simulink model "db5_2_Level_double"  (R2021a)
settings: Solver=VariableStepAuto  StartTime=0.0  StopTime=8  RelTol=1e-3
undefined symbols (not defined in the file): lambda2
libraries: dspsigops x5, dspquant2 x1
(part 1 of 2)
settings Model: Creator=Ruth Matienzo  LastModifiedBy=Ruth Matienzo

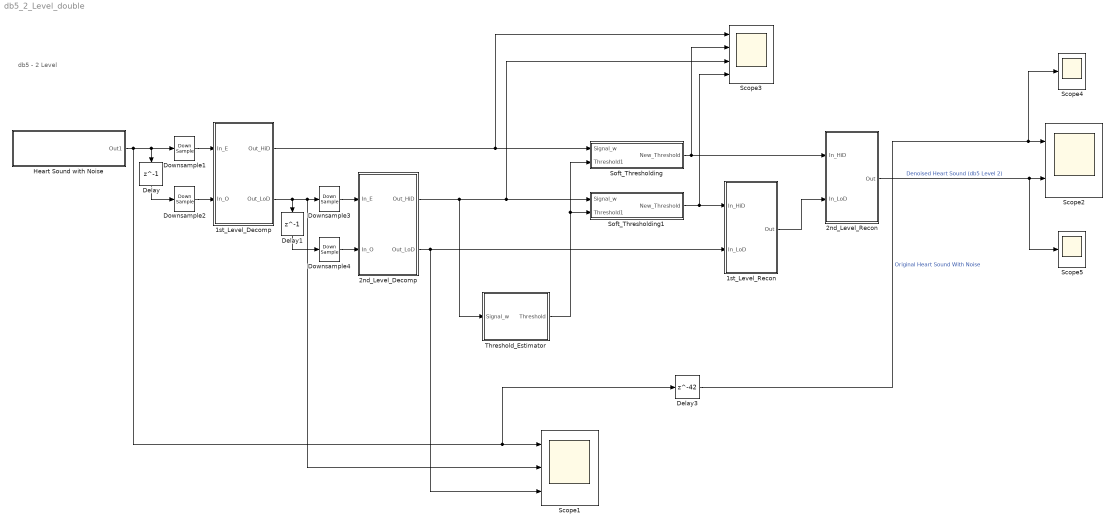
== system db5_2_Level_double ==
  note: db5 - 2 Level
  1st_Level_Decomp : Subsystem
  1st_Level_Recon : Subsystem
  2nd_Level_Decomp : Subsystem
  2nd_Level_Recon : Subsystem
  Delay : Delay  DelayLength=1  SampleTime=1/44100
  Delay1 : Delay  DelayLength=1  SampleTime=1/44100
  Delay3 : Delay  DelayLength=42  SampleTime=1/44100
  Downsample{1..4} (4 alike) : DownSample  N=30
  Heart Sound with Noise : Subsystem
  Scope1 : Scope  NumInputPorts=3
  Scope2 : Scope  NumInputPorts=2
  Scope3 : Scope  NumInputPorts=4
  Scope4 : Scope
  Scope5 : Scope
  Soft_Thresholding : Subsystem
  Soft_Thresholding1 : Subsystem
  Threshold_Estimator : Subsystem
  wires:
  1st_Level_Decomp/1(Out_HiD) -> Scope3/1, Soft_Thresholding/1(Signal_w)
  1st_Level_Recon/1(Out) -> 2nd_Level_Recon/2(In_LoD)
  Soft_Thresholding1/1(New_Threshold) -> 1st_Level_Recon/1(In_HiD), Scope3/4
  2nd_Level_Decomp/2(Out_LoD) -> 1st_Level_Recon/2(In_LoD), Scope1/3
  Downsample3/1 -> 2nd_Level_Decomp/1(In_E)
  2nd_Level_Decomp/1(Out_HiD) -> Threshold_Estimator/1(Signal_w), Scope3/3, Soft_Thresholding1/1(Signal_w)
  Downsample2/1 -> 1st_Level_Decomp/2(In_O)
  Delay1/1 -> Downsample4/1
  Heart Sound with Noise/1(Out1) -> Delay3/1, Scope1/1, Downsample1/1, Delay/1
  Downsample4/1 -> 2nd_Level_Decomp/2(In_O)
  Threshold_Estimator/1(Threshold) -> Soft_Thresholding1/2(Threshold1), Soft_Thresholding/2(Threshold1)
  Soft_Thresholding/1(New_Threshold) -> 2nd_Level_Recon/1(In_HiD), Scope3/2
  1st_Level_Decomp/2(Out_LoD) -> Scope1/2, Downsample3/1, Delay1/1
  Delay/1 -> Downsample2/1
  Downsample1/1 -> 1st_Level_Decomp/1(In_E)
  2nd_Level_Recon/1(Out) -> Scope5/1, Scope2/2  "Denoised Heart Sound (db5 Level 2)"
  Delay3/1 -> Scope4/1, Scope2/1  "Original Heart Sound With Noise"

== system db5_2_Level_double/1st_Level_Decomp ==
  In_E : Inport  OutDataTypeStr=double  SampleTime=1/44100
  In_O : Inport  Port=2  OutDataTypeStr=double  SampleTime=1/44100
  Add : Sum  AccumDataTypeStr=double  OutDataTypeStr=double
  Add1 : Sum  AccumDataTypeStr=double  OutDataTypeStr=double
  Delay1 : Delay  DelayLength=1  SampleTime=1/44100
  Delay2 : Delay  DelayLength=1  SampleTime=1/44100
  Divide1 : Product  Inputs=*/  OutDataTypeStr=double
  Divide2 : Product  Inputs=*/  OutDataTypeStr=double
  HiD : Constant  Value=1.216858059+0.784079501  OutDataTypeStr=double  SampleTime=1/44100
  HiD_Even : Subsystem
  HiD_Odd : Subsystem
  LoD : Constant  Value=0.784079501+1.216858059  OutDataTypeStr=double  SampleTime=1/44100
  LoD_Even : Subsystem
  LoD_Odd : Subsystem
  Out_HiD : Outport  OutDataTypeStr=double  SampleTime=1/44100
  Out_LoD : Outport  Port=2  OutDataTypeStr=double  SampleTime=1/44100
  wires:
  HiD/1 -> Divide1/2
  Add1/1 -> Divide2/1
  LoD/1 -> Divide2/2
  Add/1 -> Divide1/1
  Delay1/1 -> Out_HiD/1
  Divide1/1 -> Delay1/1
  Delay2/1 -> Out_LoD/1
  Divide2/1 -> Delay2/1
  In_E/1 -> LoD_Even/1(In_HiD_e), HiD_Even/1(In_HiD_e)
  HiD_Even/1(Out_HiD_e) -> Add/1
  In_O/1 -> LoD_Odd/1(In_HiD_e), HiD_Odd/1(In_HiD_e)
  HiD_Odd/1(Out_HiD_e) -> Add/2
  LoD_Even/1(Out_HiD_e) -> Add1/1
  LoD_Odd/1(Out_HiD_e) -> Add1/2

== system db5_2_Level_double/1st_Level_Recon ==
  In_HiD : Inport  OutDataTypeStr=double  SampleTime=1/44100
  In_LoD : Inport  Port=2  OutDataTypeStr=double  SampleTime=1/44100
  Add : Sum  AccumDataTypeStr=double  OutDataTypeStr=double
  Add1 : Sum  AccumDataTypeStr=double  OutDataTypeStr=double
  Add2 : Sum  AccumDataTypeStr=double  OutDataTypeStr=double
  Delay1 : Delay  DelayLength=1  SampleTime=1/44100
  Delay2 : Delay  DelayLength=1  SampleTime=1/44100
  Divide2 : Product  Inputs=*/  OutDataTypeStr=double  RndMeth=Zero  SaturateOnIntegerOverflow=on
  HiD1 : Constant  Value=0.707106781*1.41355  OutDataTypeStr=double  SampleTime=1/44100
  HiR_Even : Subsystem
  HiR_Odd : Subsystem
  LoR_Even : Subsystem
  LoR_Odd : Subsystem
  Rate Transition{,1..3} (4 alike) : RateTransition  OutPortSampleTime=1/44100
  Upsample : dspsigops/Upsample  N=30  phase=0  RateOptions=Allow multirate processing  ic=0  mode=Unused parameter value
  Upsample1 : dspsigops/Upsample  N=30  phase=0  RateOptions=Allow multirate processing  ic=0  mode=Unused parameter value
  Out : Outport  OutDataTypeStr=double  SampleTime=1/44100
  wires:
  In_HiD/1 -> HiR_Odd/1(In_HiR_o), HiR_Even/1(In_HiR_e)
  Add/1 -> Upsample1/1
  Add1/1 -> Upsample/1
  Upsample/1 -> Rate Transition/1
  Upsample1/1 -> Add2/1
  Delay2/1 -> Rate Transition1/1
  HiR_Even/1(Out_HiR_e) -> Add/1
  Rate Transition/1 -> Delay2/1
  Rate Transition1/1 -> Add2/2
  Rate Transition2/1 -> Delay1/1
  Delay1/1 -> Out/1
  HiD1/1 -> Rate Transition3/1
  Add2/1 -> Divide2/1
  Divide2/1 -> Rate Transition2/1
  Rate Transition3/1 -> Divide2/2
  In_LoD/1 -> LoR_Odd/1(In_LoR_o), LoR_Even/1(In_LoR_e)
  LoR_Even/1(Out_LoR_e) -> Add/2
  HiR_Odd/1(Out_HiR_o) -> Add1/1
  LoR_Odd/1(Out_LoR_o) -> Add1/2

== system db5_2_Level_double/2nd_Level_Decomp ==
  In_E : Inport  OutDataTypeStr=double  SampleTime=1/44100
  In_O : Inport  Port=2  OutDataTypeStr=double  SampleTime=1/44100
  Add : Sum  AccumDataTypeStr=double  OutDataTypeStr=double
  Add1 : Sum  AccumDataTypeStr=double  OutDataTypeStr=double
  Delay1 : Delay  DelayLength=1  SampleTime=1/44100
  Delay2 : Delay  DelayLength=1  SampleTime=1/44100
  Divide1 : Product  Inputs=*/  OutDataTypeStr=double
  Divide2 : Product  Inputs=*/  OutDataTypeStr=double
  HiD : Constant  Value=1.216858059+0.784079501  OutDataTypeStr=double  SampleTime=1/44100
  HiD_Even : Subsystem
  HiD_Odd : Subsystem
  LoD : Constant  Value=0.784079501+1.216858059  OutDataTypeStr=double  SampleTime=1/44100
  LoD_Even : Subsystem
  LoD_Odd : Subsystem
  Out_HiD : Outport  OutDataTypeStr=double  SampleTime=1/44100
  Out_LoD : Outport  Port=2  OutDataTypeStr=double  SampleTime=1/44100
  wires:
  HiD/1 -> Divide1/2
  Add1/1 -> Divide2/1
  LoD/1 -> Divide2/2
  Add/1 -> Divide1/1
  Delay1/1 -> Out_HiD/1
  Divide1/1 -> Delay1/1
  Delay2/1 -> Out_LoD/1
  Divide2/1 -> Delay2/1
  In_E/1 -> LoD_Even/1(In_HiD_e), HiD_Even/1(In_HiD_e)
  HiD_Even/1(Out_HiD_e) -> Add/1
  In_O/1 -> LoD_Odd/1(In_HiD_e), HiD_Odd/1(In_HiD_e)
  HiD_Odd/1(Out_HiD_e) -> Add/2
  LoD_Even/1(Out_HiD_e) -> Add1/1
  LoD_Odd/1(Out_HiD_e) -> Add1/2

== system db5_2_Level_double/2nd_Level_Recon ==
  In_HiD : Inport  OutDataTypeStr=double  SampleTime=1/44100
  In_LoD : Inport  Port=2  OutDataTypeStr=double  SampleTime=1/44100
  Add : Sum  AccumDataTypeStr=double  OutDataTypeStr=double
  Add1 : Sum  AccumDataTypeStr=double  OutDataTypeStr=double
  Add2 : Sum  AccumDataTypeStr=double  OutDataTypeStr=double
  Delay1 : Delay  DelayLength=1  SampleTime=1/44100
  Delay2 : Delay  DelayLength=1  SampleTime=1/44100
  Divide2 : Product  Inputs=*/  OutDataTypeStr=double  RndMeth=Zero  SaturateOnIntegerOverflow=on
  HiD1 : Constant  Value=0.707106781*1.41355  OutDataTypeStr=double  SampleTime=1/44100
  HiR_Even : Subsystem
  HiR_Odd : Subsystem
  LoR_Even : Subsystem
  LoR_Odd : Subsystem
  Rate Transition{,1..3} (4 alike) : RateTransition  OutPortSampleTime=1/44100
  Upsample : dspsigops/Upsample  N=30  phase=0  RateOptions=Allow multirate processing  ic=0  mode=Unused parameter value
  Upsample1 : dspsigops/Upsample  N=30  phase=0  RateOptions=Allow multirate processing  ic=0  mode=Unused parameter value
  Out : Outport  OutDataTypeStr=double  SampleTime=1/44100
  wires:
  In_HiD/1 -> HiR_Odd/1(In_HiR_o), HiR_Even/1(In_HiR_e)
  Add/1 -> Upsample1/1
  Add1/1 -> Upsample/1
  Upsample/1 -> Rate Transition/1
  Upsample1/1 -> Add2/1
  Delay2/1 -> Rate Transition1/1
  HiR_Even/1(Out_HiR_e) -> Add/1
  Rate Transition/1 -> Delay2/1
  Rate Transition1/1 -> Add2/2
  Rate Transition2/1 -> Delay1/1
  Delay1/1 -> Out/1
  HiD1/1 -> Rate Transition3/1
  Add2/1 -> Divide2/1
  Divide2/1 -> Rate Transition2/1
  Rate Transition3/1 -> Divide2/2
  In_LoD/1 -> LoR_Odd/1(In_LoR_o), LoR_Even/1(In_LoR_e)
  LoR_Even/1(Out_LoR_e) -> Add/2
  HiR_Odd/1(Out_HiR_o) -> Add1/1
  LoR_Odd/1(Out_LoR_o) -> Add1/2

== system db5_2_Level_double/Heart Sound with Noise ==
  Constant : Constant  Value=80000  OutDataTypeStr=double  SampleTime=1/44100
  Divide : Product  Inputs=*/  OutDataTypeStr=double
  From Workspace1 : FromWorkspace  VariableName=Audio_Heart_Noise  OutDataTypeStr=double  SampleTime=1/44100
  Gain2 : Gain  Gain=5  ParamDataTypeStr=double  OutDataTypeStr=double
  Pulse Generator : DiscretePulseGenerator  PulseType=Time based  Period=0.00022675736  PulseWidth=50
  Quantizer : Quantizer  QuantizationInterval=0.1
  Sample and Hold : dspsigops/Sample and Hold  trig=Rising edge  initCond=0  latchinput=off
  Uniform Encoder : dspquant2/Uniform Encoder  peak=2  bits=8  otype=Unsigned integer
  Out1 : Outport  OutDataTypeStr=double  SampleTime=1/44100
  wires:
  Sample and Hold/1 -> Quantizer/1
  Uniform Encoder/1 -> Divide/1
  Quantizer/1 -> Uniform Encoder/1
  Constant/1 -> Divide/2
  From Workspace1/1 -> Gain2/1
  Pulse Generator/1 -> Sample and Hold/Trigger
  Gain2/1 -> Sample and Hold/1
  Divide/1 -> Out1/1

== system db5_2_Level_double/Soft_Thresholding ==
  Signal_w : Inport  OutDataTypeStr=double  SampleTime=1/44100
  Threshold1 : Inport  Port=2  OutDataTypeStr=double  SampleTime=1/44100
  Abs : Abs  OutDataTypeStr=double
  Add1 : Sum  AccumDataTypeStr=double  OutDataTypeStr=double
  Constant : Constant  Value=0  OutDataTypeStr=double  SampleTime=1/44100
  Delay{1..7} (7 alike) : Delay  DelayLength=1  SampleTime=1/44100
  Divide : Product  Inputs=*/  OutDataTypeStr=double
  Gain1 : Gain  Gain=-1  ParamDataTypeStr=double  OutMin=-1  OutMax=-0.99  OutDataTypeStr=double
  Length : Constant  Value=lambda2  OutDataTypeStr=double  SampleTime=1/44100
  Relational Operator1 : RelationalOperator  Operator===  OutDataTypeStr=boolean  RndMeth=Simplest
  Relational Operator2 : RelationalOperator  Operator=>  OutDataTypeStr=boolean  RndMeth=Simplest
  Relational Operator3 : RelationalOperator  Operator=<  OutDataTypeStr=boolean  RndMeth=Simplest
  Relational Operator4 : RelationalOperator  Operator=>  OutDataTypeStr=boolean  RndMeth=Simplest
  Relational Operator5 : RelationalOperator  Operator=<  OutDataTypeStr=boolean  RndMeth=Simplest
  Relational Operator6 : RelationalOperator  Operator=>  OutDataTypeStr=boolean  RndMeth=Simplest
  Relational Operator7 : RelationalOperator  Operator===  OutDataTypeStr=boolean  RndMeth=Simplest
  Subtract1 : Sum  Inputs=+-  AccumDataTypeStr=double  OutDataTypeStr=double
  Threshold_Switch : Switch  Threshold=1  OutDataTypeStr=double
  Threshold_Switch1 : Switch  Threshold=1  OutDataTypeStr=double
  Threshold_Switch2 : Switch  Threshold=1  OutDataTypeStr=double
  New_Threshold : Outport  OutDataTypeStr=double  SampleTime=1/44100
  wires:
  Threshold_Switch/1 -> Threshold_Switch2/3
  Relational Operator6/1 -> Threshold_Switch1/2
  Gain1/1 -> Relational Operator3/2
  Delay4/1 -> Threshold_Switch/3
  Add1/1 -> Delay4/1
  Delay2/1 -> Relational Operator4/1
  Delay3/1 -> Relational Operator4/2
  Delay1/1 -> Threshold_Switch/1
  Relational Operator2/1 -> Delay2/1
  Relational Operator3/1 -> Delay3/1
  Relational Operator5/1 -> Delay6/1
  Delay6/1 -> Relational Operator6/2
  Delay5/1 -> Relational Operator6/1
  Threshold1/1 -> Relational Operator2/2, Subtract1/2, Relational Operator5/2, Relational Operator1/2, Add1/2, Gain1/1, Relational Operator7/2
  Abs/1 -> Relational Operator1/1
  Relational Operator4/1 -> Threshold_Switch/2
  Subtract1/1 -> Delay1/1
  Constant/1 -> Threshold_Switch1/3, Threshold_Switch1/1
  Signal_w/1 -> Subtract1/1, Relational Operator2/1, Relational Operator5/1, Abs/1, Add1/1, Relational Operator3/1, Relational Operator7/1
  Relational Operator7/1 -> Threshold_Switch2/2
  Relational Operator1/1 -> Delay5/1
  Threshold_Switch1/1 -> Threshold_Switch2/1
  Threshold_Switch2/1 -> Divide/1
  Length/1 -> Divide/2
  Divide/1 -> Delay7/1
  Delay7/1 -> New_Threshold/1

== system db5_2_Level_double/Soft_Thresholding1 ==
  Signal_w : Inport  OutDataTypeStr=double  SampleTime=1/44100
  Threshold1 : Inport  Port=2  OutDataTypeStr=double  SampleTime=1/44100
  Abs : Abs  OutDataTypeStr=double
  Add1 : Sum  AccumDataTypeStr=double  OutDataTypeStr=double
  Constant : Constant  Value=0  OutDataTypeStr=double  SampleTime=1/44100
  Delay{1..7} (7 alike) : Delay  DelayLength=1  SampleTime=1/44100
  Divide : Product  Inputs=*/  OutDataTypeStr=double
  Gain1 : Gain  Gain=-1  ParamDataTypeStr=double  OutMin=-1  OutMax=-0.99  OutDataTypeStr=double
  Length : Constant  Value=lambda2  OutDataTypeStr=double  SampleTime=1/44100
  Relational Operator1 : RelationalOperator  Operator===  OutDataTypeStr=boolean  RndMeth=Simplest
  Relational Operator2 : RelationalOperator  Operator=>  OutDataTypeStr=boolean  RndMeth=Simplest
  Relational Operator3 : RelationalOperator  Operator=<  OutDataTypeStr=boolean  RndMeth=Simplest
  Relational Operator4 : RelationalOperator  Operator=>  OutDataTypeStr=boolean  RndMeth=Simplest
  Relational Operator5 : RelationalOperator  Operator=<  OutDataTypeStr=boolean  RndMeth=Simplest
  Relational Operator6 : RelationalOperator  Operator=>  OutDataTypeStr=boolean  RndMeth=Simplest
  Relational Operator7 : RelationalOperator  Operator===  OutDataTypeStr=boolean  RndMeth=Simplest
  Subtract1 : Sum  Inputs=+-  AccumDataTypeStr=double  OutDataTypeStr=double
  Threshold_Switch : Switch  Threshold=1  OutDataTypeStr=double
  Threshold_Switch1 : Switch  Threshold=1  OutDataTypeStr=double
  Threshold_Switch2 : Switch  Threshold=1  OutDataTypeStr=double
  New_Threshold : Outport  OutDataTypeStr=double  SampleTime=1/44100
  wires:
  Threshold_Switch/1 -> Threshold_Switch2/3
  Relational Operator6/1 -> Threshold_Switch1/2
  Gain1/1 -> Relational Operator3/2
  Delay4/1 -> Threshold_Switch/3
  Add1/1 -> Delay4/1
  Delay2/1 -> Relational Operator4/1
  Delay3/1 -> Relational Operator4/2
  Delay1/1 -> Threshold_Switch/1
  Relational Operator2/1 -> Delay2/1
  Relational Operator3/1 -> Delay3/1
  Relational Operator5/1 -> Delay6/1
  Delay6/1 -> Relational Operator6/2
  Delay5/1 -> Relational Operator6/1
  Threshold1/1 -> Relational Operator2/2, Subtract1/2, Relational Operator5/2, Relational Operator1/2, Add1/2, Gain1/1, Relational Operator7/2
  Abs/1 -> Relational Operator1/1
  Relational Operator4/1 -> Threshold_Switch/2
  Subtract1/1 -> Delay1/1
  Constant/1 -> Threshold_Switch1/3, Threshold_Switch1/1
  Signal_w/1 -> Subtract1/1, Relational Operator2/1, Relational Operator5/1, Abs/1, Add1/1, Relational Operator3/1, Relational Operator7/1
  Relational Operator7/1 -> Threshold_Switch2/2
  Relational Operator1/1 -> Delay5/1
  Threshold_Switch1/1 -> Threshold_Switch2/1
  Threshold_Switch2/1 -> Divide/1
  Length/1 -> Divide/2
  Divide/1 -> Delay7/1
  Delay7/1 -> New_Threshold/1

== system db5_2_Level_double/Threshold_Estimator ==
  Signal_w : Inport  OutDataTypeStr=double  SampleTime=1/44100
  Absolute_Value1 : Subsystem
  Length : Constant  Value=lambda2  OutDataTypeStr=double  SampleTime=1/44100
  Median2 : Subsystem
  Multiply : Product  OutDataTypeStr=double
  Threshold : Outport  OutDataTypeStr=double  SampleTime=1/44100  VectorParamsAs1DForOutWhenUnconnected=off
  wires:
  Length/1 -> Multiply/2
  Median2/1(Median) -> Multiply/1
  Absolute_Value1/1(Out_Abs) -> Median2/1(Signal_w3)
  Signal_w/1 -> Absolute_Value1/1(Signal_w4)
  Multiply/1 -> Threshold/1

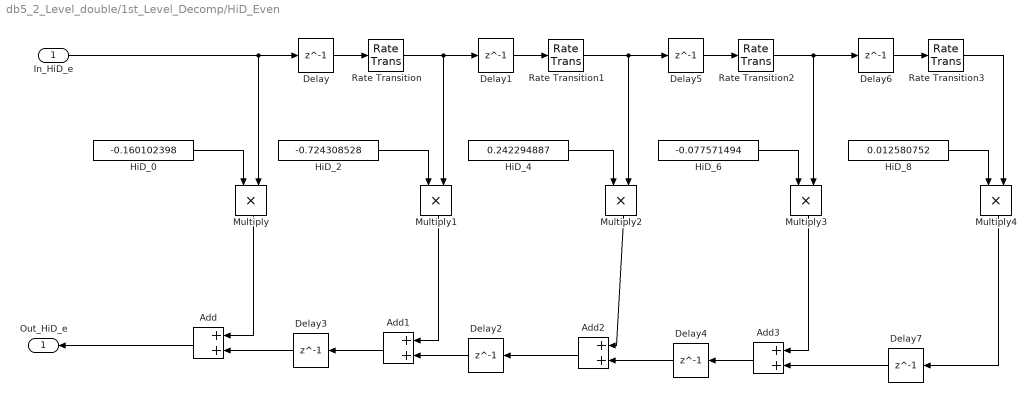
== system db5_2_Level_double/1st_Level_Decomp/HiD_Even ==
  In_HiD_e : Inport  OutDataTypeStr=double  SampleTime=1/44100
  Add{,1..3} (4 alike) : Sum  AccumDataTypeStr=double  OutDataTypeStr=double
  Delay{,1..7} (8 alike) : Delay  DelayLength=1  SampleTime=1/44100
  HiD_0 : Constant  Value=-0.160102398  OutDataTypeStr=double  SampleTime=1/44100
  HiD_2 : Constant  Value=-0.724308528  OutDataTypeStr=double  SampleTime=1/44100
  HiD_4 : Constant  Value=0.242294887  OutDataTypeStr=double  SampleTime=1/44100
  HiD_6 : Constant  Value=-0.077571494  OutDataTypeStr=double  SampleTime=1/44100
  HiD_8 : Constant  Value=0.012580752  OutDataTypeStr=double  SampleTime=1/44100
  Multiply{,1..4} (5 alike) : Product  OutDataTypeStr=double
  Rate Transition{,1..3} (4 alike) : RateTransition  OutPortSampleTime=1/44100
  Out_HiD_e : Outport  OutDataTypeStr=double  SampleTime=1/44100  VectorParamsAs1DForOutWhenUnconnected=off
  wires:
  Delay1/1 -> Rate Transition1/1
  Delay3/1 -> Add/2
  HiD_2/1 -> Multiply1/1
  Rate Transition2/1 -> Delay6/1, Multiply3/2
  Add/1 -> Out_HiD_e/1
  Delay4/1 -> Add2/2
  Delay5/1 -> Rate Transition2/1
  Rate Transition1/1 -> Delay5/1, Multiply2/2
  HiD_0/1 -> Multiply/1
  Multiply2/1 -> Add2/1
  Add2/1 -> Delay2/1
  HiD_6/1 -> Multiply3/1
  Multiply/1 -> Add/1
  In_HiD_e/1 -> Delay/1, Multiply/2
  Multiply1/1 -> Add1/1
  Rate Transition/1 -> Delay1/1, Multiply1/2
  Add1/1 -> Delay3/1
  HiD_4/1 -> Multiply2/1
  Delay/1 -> Rate Transition/1
  Delay2/1 -> Add1/2
  HiD_8/1 -> Multiply4/1
  Delay6/1 -> Rate Transition3/1
  Rate Transition3/1 -> Multiply4/2
  Multiply4/1 -> Delay7/1
  Multiply3/1 -> Add3/1
  Add3/1 -> Delay4/1
  Delay7/1 -> Add3/2

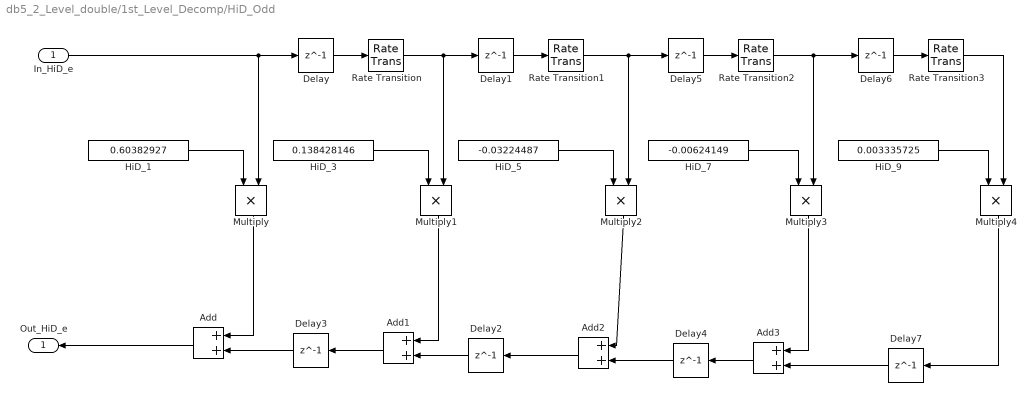
== system db5_2_Level_double/1st_Level_Decomp/HiD_Odd ==
  In_HiD_e : Inport  OutDataTypeStr=double  SampleTime=1/44100
  Add{,1..3} (4 alike) : Sum  AccumDataTypeStr=double  OutDataTypeStr=double
  Delay{,1..7} (8 alike) : Delay  DelayLength=1  SampleTime=1/44100
  HiD_1 : Constant  Value=0.60382927  OutDataTypeStr=double  SampleTime=1/44100
  HiD_3 : Constant  Value=0.138428146  OutDataTypeStr=double  SampleTime=1/44100
  HiD_5 : Constant  Value=-0.03224487  OutDataTypeStr=double  SampleTime=1/44100
  HiD_7 : Constant  Value=-0.00624149  OutDataTypeStr=double  SampleTime=1/44100
  HiD_9 : Constant  Value=0.003335725  OutDataTypeStr=double  SampleTime=1/44100
  Multiply{,1..4} (5 alike) : Product  OutDataTypeStr=double
  Rate Transition{,1..3} (4 alike) : RateTransition  OutPortSampleTime=1/44100
  Out_HiD_e : Outport  OutDataTypeStr=double  SampleTime=1/44100  VectorParamsAs1DForOutWhenUnconnected=off
  wires:
  Multiply4/1 -> Delay7/1
  Delay6/1 -> Rate Transition3/1
  Rate Transition3/1 -> Multiply4/2
  Add3/1 -> Delay4/1
  Add/1 -> Out_HiD_e/1
  Delay1/1 -> Rate Transition1/1
  Delay7/1 -> Add3/2
  Rate Transition2/1 -> Delay6/1, Multiply3/2
  Delay3/1 -> Add/2
  Rate Transition/1 -> Delay1/1, Multiply1/2
  Rate Transition1/1 -> Delay5/1, Multiply2/2
  Delay4/1 -> Add2/2
  Multiply/1 -> Add/1
  Add2/1 -> Delay2/1
  Delay5/1 -> Rate Transition2/1
  Multiply1/1 -> Add1/1
  Delay2/1 -> Add1/2
  Delay/1 -> Rate Transition/1
  Add1/1 -> Delay3/1
  Multiply3/1 -> Add3/1
  HiD_3/1 -> Multiply1/1
  Multiply2/1 -> Add2/1
  HiD_7/1 -> Multiply3/1
  In_HiD_e/1 -> Delay/1, Multiply/2
  HiD_1/1 -> Multiply/1
  HiD_5/1 -> Multiply2/1
  HiD_9/1 -> Multiply4/1

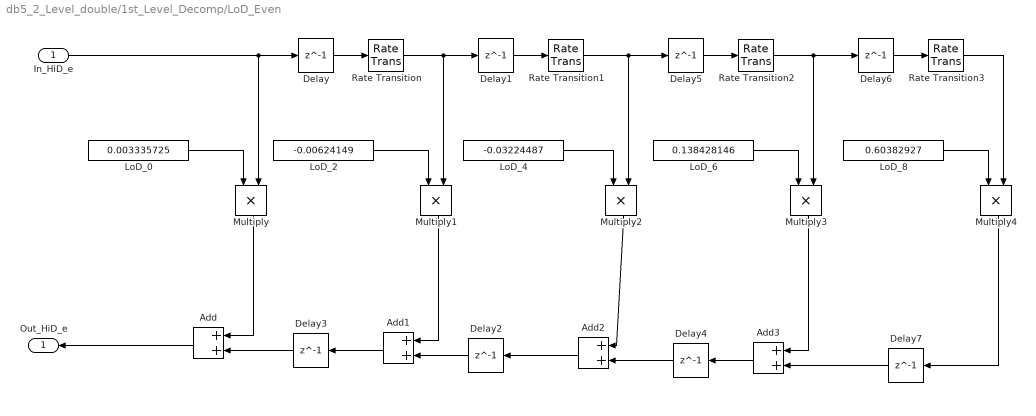
== system db5_2_Level_double/1st_Level_Decomp/LoD_Even ==
  In_HiD_e : Inport  OutDataTypeStr=double  SampleTime=1/44100
  Add{,1..3} (4 alike) : Sum  AccumDataTypeStr=double  OutDataTypeStr=double
  Delay{,1..7} (8 alike) : Delay  DelayLength=1  SampleTime=1/44100
  LoD_0 : Constant  Value=0.003335725  OutDataTypeStr=double  SampleTime=1/44100
  LoD_2 : Constant  Value=-0.00624149  OutDataTypeStr=double  SampleTime=1/44100
  LoD_4 : Constant  Value=-0.03224487  OutDataTypeStr=double  SampleTime=1/44100
  LoD_6 : Constant  Value=0.138428146  OutDataTypeStr=double  SampleTime=1/44100
  LoD_8 : Constant  Value=0.60382927  OutDataTypeStr=double  SampleTime=1/44100
  Multiply{,1..4} (5 alike) : Product  OutDataTypeStr=double
  Rate Transition{,1..3} (4 alike) : RateTransition  OutPortSampleTime=1/44100
  Out_HiD_e : Outport  OutDataTypeStr=double  SampleTime=1/44100  VectorParamsAs1DForOutWhenUnconnected=off
  wires:
  Multiply3/1 -> Add3/1
  LoD_4/1 -> Multiply2/1
  Multiply2/1 -> Add2/1
  Add1/1 -> Delay3/1
  Delay2/1 -> Add1/2
  Delay/1 -> Rate Transition/1
  Multiply1/1 -> Add1/1
  In_HiD_e/1 -> Delay/1, Multiply/2
  Add2/1 -> Delay2/1
  Delay5/1 -> Rate Transition2/1
  Multiply/1 -> Add/1
  LoD_8/1 -> Multiply4/1
  Delay4/1 -> Add2/2
  Rate Transition1/1 -> Delay5/1, Multiply2/2
  Rate Transition/1 -> Delay1/1, Multiply1/2
  Delay3/1 -> Add/2
  Rate Transition2/1 -> Delay6/1, Multiply3/2
  Add/1 -> Out_HiD_e/1
  Delay1/1 -> Rate Transition1/1
  Delay7/1 -> Add3/2
  LoD_6/1 -> Multiply3/1
  Add3/1 -> Delay4/1
  Rate Transition3/1 -> Multiply4/2
  Delay6/1 -> Rate Transition3/1
  Multiply4/1 -> Delay7/1
  LoD_2/1 -> Multiply1/1
  LoD_0/1 -> Multiply/1

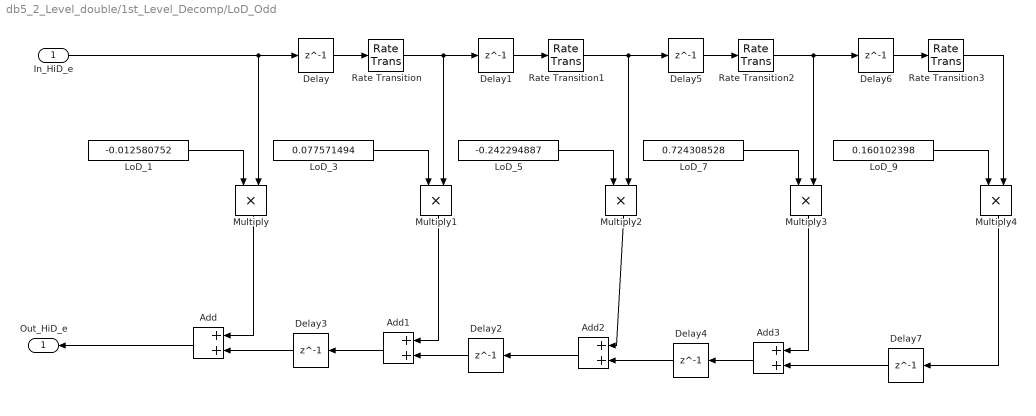
== system db5_2_Level_double/1st_Level_Decomp/LoD_Odd ==
  In_HiD_e : Inport  OutDataTypeStr=double  SampleTime=1/44100
  Add{,1..3} (4 alike) : Sum  AccumDataTypeStr=double  OutDataTypeStr=double
  Delay{,1..7} (8 alike) : Delay  DelayLength=1  SampleTime=1/44100
  LoD_1 : Constant  Value=-0.012580752  OutDataTypeStr=double  SampleTime=1/44100
  LoD_3 : Constant  Value=0.077571494  OutDataTypeStr=double  SampleTime=1/44100
  LoD_5 : Constant  Value=-0.242294887  OutDataTypeStr=double  SampleTime=1/44100
  LoD_7 : Constant  Value=0.724308528  OutDataTypeStr=double  SampleTime=1/44100
  LoD_9 : Constant  Value=0.160102398  OutDataTypeStr=double  SampleTime=1/44100
  Multiply{,1..4} (5 alike) : Product  OutDataTypeStr=double
  Rate Transition{,1..3} (4 alike) : RateTransition  OutPortSampleTime=1/44100
  Out_HiD_e : Outport  OutDataTypeStr=double  SampleTime=1/44100  VectorParamsAs1DForOutWhenUnconnected=off
  wires:
  LoD_9/1 -> Multiply4/1
  LoD_3/1 -> Multiply1/1
  LoD_5/1 -> Multiply2/1
  In_HiD_e/1 -> Delay/1, Multiply/2
  LoD_1/1 -> Multiply/1
  Multiply1/1 -> Add1/1
  Multiply3/1 -> Add3/1
  Multiply2/1 -> Add2/1
  Add1/1 -> Delay3/1
  Delay2/1 -> Add1/2
  Delay5/1 -> Rate Transition2/1
  Rate Transition/1 -> Delay1/1, Multiply1/2
  Multiply/1 -> Add/1
  Add2/1 -> Delay2/1
  Delay/1 -> Rate Transition/1
  Delay4/1 -> Add2/2
  Delay3/1 -> Add/2
  Delay7/1 -> Add3/2
  Add/1 -> Out_HiD_e/1
  Delay1/1 -> Rate Transition1/1
  Rate Transition2/1 -> Delay6/1, Multiply3/2
  Rate Transition1/1 -> Delay5/1, Multiply2/2
  LoD_7/1 -> Multiply3/1
  Multiply4/1 -> Delay7/1
  Delay6/1 -> Rate Transition3/1
  Add3/1 -> Delay4/1
  Rate Transition3/1 -> Multiply4/2

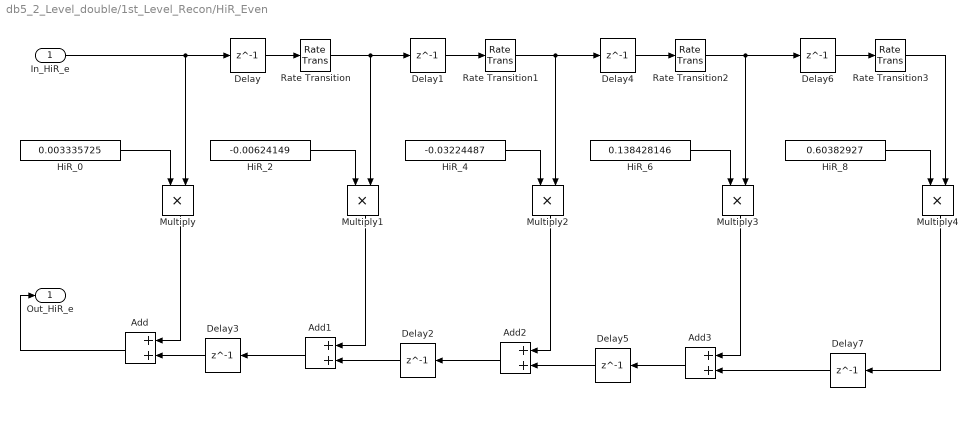
== system db5_2_Level_double/1st_Level_Recon/HiR_Even ==
  In_HiR_e : Inport  OutDataTypeStr=double  SampleTime=1/44100
  Add{,1..3} (4 alike) : Sum  AccumDataTypeStr=double  OutDataTypeStr=double
  Delay{,1..7} (8 alike) : Delay  DelayLength=1  SampleTime=1/44100
  HiR_0 : Constant  Value=0.003335725  OutDataTypeStr=double  SampleTime=1/44100
  HiR_2 : Constant  Value=-0.00624149  OutDataTypeStr=double  SampleTime=1/44100
  HiR_4 : Constant  Value=-0.03224487  OutDataTypeStr=double  SampleTime=1/44100
  HiR_6 : Constant  Value=0.138428146  OutDataTypeStr=double  SampleTime=1/44100
  HiR_8 : Constant  Value=0.60382927  OutDataTypeStr=double  SampleTime=1/44100
  Multiply{,1..4} (5 alike) : Product  OutDataTypeStr=double
  Rate Transition{,1..3} (4 alike) : RateTransition  OutPortSampleTime=1/44100
  Out_HiR_e : Outport  OutDataTypeStr=double  SampleTime=1/44100  VectorParamsAs1DForOutWhenUnconnected=off
  wires:
  Delay3/1 -> Add/2
  In_HiR_e/1 -> Delay/1, Multiply/2
  HiR_4/1 -> Multiply2/1
  Multiply/1 -> Add/1
  Add1/1 -> Delay3/1
  Multiply1/1 -> Add1/1
  Delay2/1 -> Add1/2
  Add/1 -> Out_HiR_e/1
  HiR_0/1 -> Multiply/1
  HiR_2/1 -> Multiply1/1
  Delay1/1 -> Rate Transition1/1
  Rate Transition/1 -> Delay1/1, Multiply1/2
  Rate Transition1/1 -> Delay4/1, Multiply2/2
  Delay/1 -> Rate Transition/1
  Delay4/1 -> Rate Transition2/1
  HiR_6/1 -> Multiply3/1
  Multiply2/1 -> Add2/1
  Add2/1 -> Delay2/1
  Delay5/1 -> Add2/2
  Rate Transition3/1 -> Multiply4/2
  Multiply4/1 -> Delay7/1
  HiR_8/1 -> Multiply4/1
  Rate Transition2/1 -> Delay6/1, Multiply3/2
  Delay6/1 -> Rate Transition3/1
  Add3/1 -> Delay5/1
  Multiply3/1 -> Add3/1
  Delay7/1 -> Add3/2

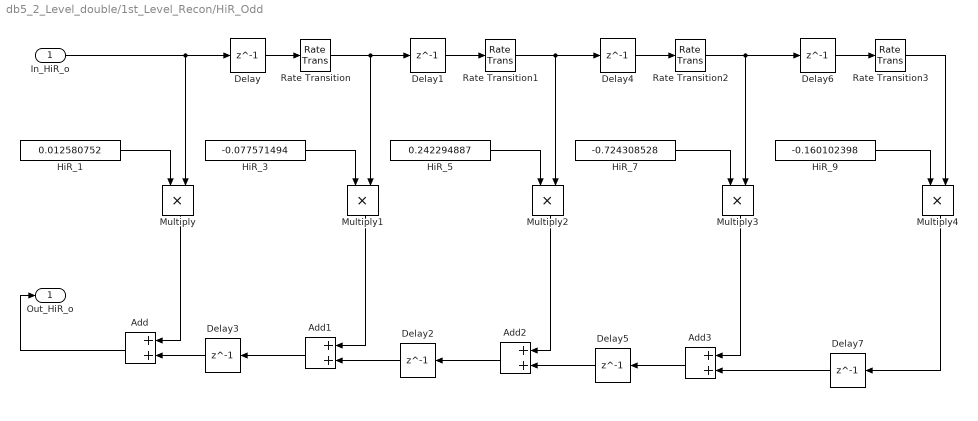
== system db5_2_Level_double/1st_Level_Recon/HiR_Odd ==
  In_HiR_o : Inport  OutDataTypeStr=double  SampleTime=1/44100
  Add{,1..3} (4 alike) : Sum  AccumDataTypeStr=double  OutDataTypeStr=double
  Delay{,1..7} (8 alike) : Delay  DelayLength=1  SampleTime=1/44100
  HiR_1 : Constant  Value=0.012580752  OutDataTypeStr=double  SampleTime=1/44100
  HiR_3 : Constant  Value=-0.077571494  OutDataTypeStr=double  SampleTime=1/44100
  HiR_5 : Constant  Value=0.242294887  OutDataTypeStr=double  SampleTime=1/44100
  HiR_7 : Constant  Value=-0.724308528  OutDataTypeStr=double  SampleTime=1/44100
  HiR_9 : Constant  Value=-0.160102398  OutDataTypeStr=double  SampleTime=1/44100
  Multiply{,1..4} (5 alike) : Product  OutDataTypeStr=double
  Rate Transition{,1..3} (4 alike) : RateTransition  OutPortSampleTime=1/44100
  Out_HiR_o : Outport  OutDataTypeStr=double  SampleTime=1/44100  VectorParamsAs1DForOutWhenUnconnected=off
  wires:
  Add/1 -> Out_HiR_o/1
  Add2/1 -> Delay2/1
  Delay5/1 -> Add2/2
  HiR_9/1 -> Multiply4/1
  HiR_5/1 -> Multiply2/1
  HiR_1/1 -> Multiply/1
  HiR_7/1 -> Multiply3/1
  Multiply1/1 -> Add1/1
  Multiply2/1 -> Add2/1
  Delay2/1 -> Add1/2
  Delay4/1 -> Rate Transition2/1
  Delay3/1 -> Add/2
  In_HiR_o/1 -> Delay/1, Multiply/2
  Rate Transition/1 -> Delay1/1, Multiply1/2
  Rate Transition2/1 -> Delay6/1, Multiply3/2
  Delay7/1 -> Add3/2
  Delay6/1 -> Rate Transition3/1
  Add3/1 -> Delay5/1
  Rate Transition3/1 -> Multiply4/2
  HiR_3/1 -> Multiply1/1
  Multiply3/1 -> Add3/1
  Add1/1 -> Delay3/1
  Multiply4/1 -> Delay7/1
  Multiply/1 -> Add/1
  Rate Transition1/1 -> Delay4/1, Multiply2/2
  Delay1/1 -> Rate Transition1/1
  Delay/1 -> Rate Transition/1

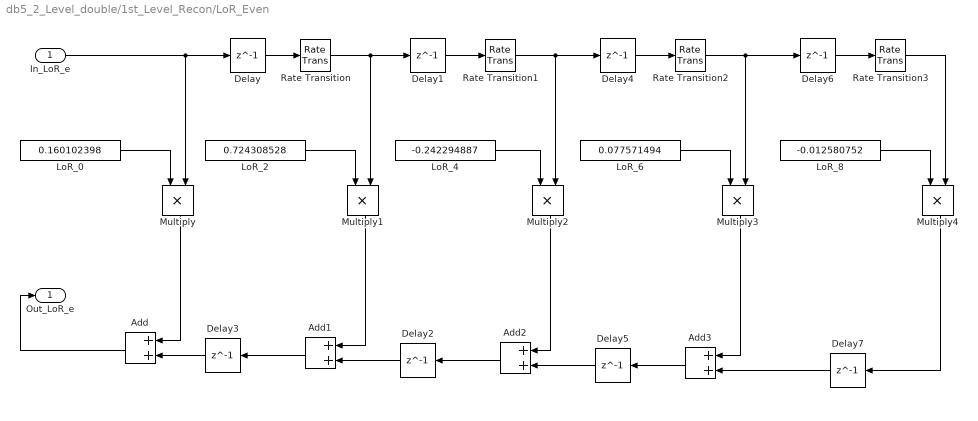
== system db5_2_Level_double/1st_Level_Recon/LoR_Even ==
  In_LoR_e : Inport  OutDataTypeStr=double  SampleTime=1/44100
  Add{,1..3} (4 alike) : Sum  AccumDataTypeStr=double  OutDataTypeStr=double
  Delay{,1..7} (8 alike) : Delay  DelayLength=1  SampleTime=1/44100
  LoR_0 : Constant  Value=0.160102398  OutDataTypeStr=double  SampleTime=1/44100
  LoR_2 : Constant  Value=0.724308528  OutDataTypeStr=double  SampleTime=1/44100
  LoR_4 : Constant  Value=-0.242294887  OutDataTypeStr=double  SampleTime=1/44100
  LoR_6 : Constant  Value=0.077571494  OutDataTypeStr=double  SampleTime=1/44100
  LoR_8 : Constant  Value=-0.012580752  OutDataTypeStr=double  SampleTime=1/44100
  Multiply{,1..4} (5 alike) : Product  OutDataTypeStr=double
  Rate Transition{,1..3} (4 alike) : RateTransition  OutPortSampleTime=1/44100
  Out_LoR_e : Outport  OutDataTypeStr=double  SampleTime=1/44100  VectorParamsAs1DForOutWhenUnconnected=off
  wires:
  Add2/1 -> Delay2/1
  Delay5/1 -> Add2/2
  Add/1 -> Out_LoR_e/1
  Delay1/1 -> Rate Transition1/1
  Rate Transition1/1 -> Delay4/1, Multiply2/2
  Multiply/1 -> Add/1
  Add1/1 -> Delay3/1
  Delay/1 -> Rate Transition/1
  Multiply2/1 -> Add2/1
  Multiply1/1 -> Add1/1
  Delay3/1 -> Add/2
  Delay4/1 -> Rate Transition2/1
  Delay2/1 -> Add1/2
  Rate Transition/1 -> Delay1/1, Multiply1/2
  In_LoR_e/1 -> Delay/1, Multiply/2
  LoR_4/1 -> Multiply2/1
  Delay6/1 -> Rate Transition3/1
  LoR_0/1 -> Multiply/1
  Delay7/1 -> Add3/2
  Rate Transition2/1 -> Delay6/1, Multiply3/2
  LoR_8/1 -> Multiply4/1
  LoR_2/1 -> Multiply1/1
  Rate Transition3/1 -> Multiply4/2
  LoR_6/1 -> Multiply3/1
  Multiply4/1 -> Delay7/1
  Multiply3/1 -> Add3/1
  Add3/1 -> Delay5/1

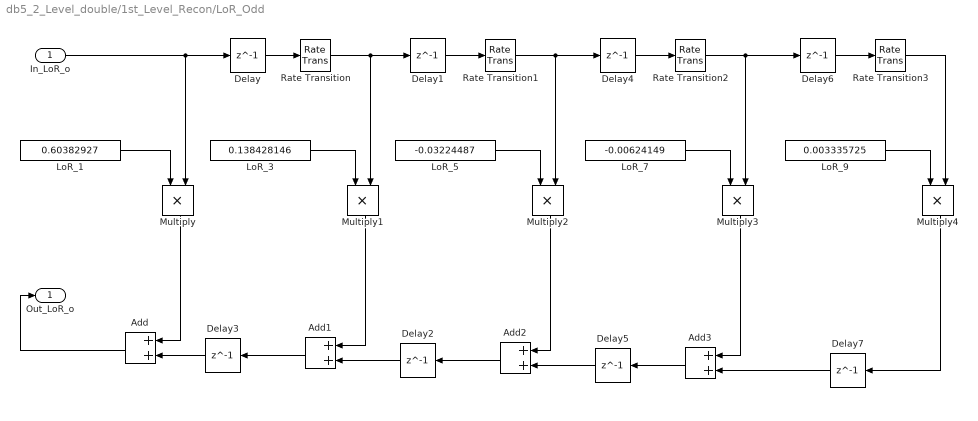
== system db5_2_Level_double/1st_Level_Recon/LoR_Odd ==
  In_LoR_o : Inport  OutDataTypeStr=double  SampleTime=1/44100
  Add{,1..3} (4 alike) : Sum  AccumDataTypeStr=double  OutDataTypeStr=double
  Delay{,1..7} (8 alike) : Delay  DelayLength=1  SampleTime=1/44100
  LoR_1 : Constant  Value=0.60382927  OutDataTypeStr=double  SampleTime=1/44100
  LoR_3 : Constant  Value=0.138428146  OutDataTypeStr=double  SampleTime=1/44100
  LoR_5 : Constant  Value=-0.03224487  OutDataTypeStr=double  SampleTime=1/44100
  LoR_7 : Constant  Value=-0.00624149  OutDataTypeStr=double  SampleTime=1/44100
  LoR_9 : Constant  Value=0.003335725  OutDataTypeStr=double  SampleTime=1/44100
  Multiply{,1..4} (5 alike) : Product  OutDataTypeStr=double
  Rate Transition{,1..3} (4 alike) : RateTransition  OutPortSampleTime=1/44100
  Out_LoR_o : Outport  OutDataTypeStr=double  SampleTime=1/44100  VectorParamsAs1DForOutWhenUnconnected=off
  wires:
  LoR_9/1 -> Multiply4/1
  Rate Transition2/1 -> Delay6/1, Multiply3/2
  Rate Transition/1 -> Delay1/1, Multiply1/2
  Rate Transition3/1 -> Multiply4/2
  Add3/1 -> Delay5/1
  Delay6/1 -> Rate Transition3/1
  Delay7/1 -> Add3/2
  LoR_1/1 -> Multiply/1
  LoR_3/1 -> Multiply1/1
  Delay3/1 -> Add/2
  Delay4/1 -> Rate Transition2/1
  LoR_5/1 -> Multiply2/1
  Delay2/1 -> Add1/2
  Multiply2/1 -> Add2/1
  Add2/1 -> Delay2/1
  LoR_7/1 -> Multiply3/1
  Delay5/1 -> Add2/2
  Multiply3/1 -> Add3/1
  Multiply/1 -> Add/1
  Delay1/1 -> Rate Transition1/1
  Multiply4/1 -> Delay7/1
  In_LoR_o/1 -> Delay/1, Multiply/2
  Add1/1 -> Delay3/1
  Add/1 -> Out_LoR_o/1
  Rate Transition1/1 -> Delay4/1, Multiply2/2
  Delay/1 -> Rate Transition/1
  Multiply1/1 -> Add1/1

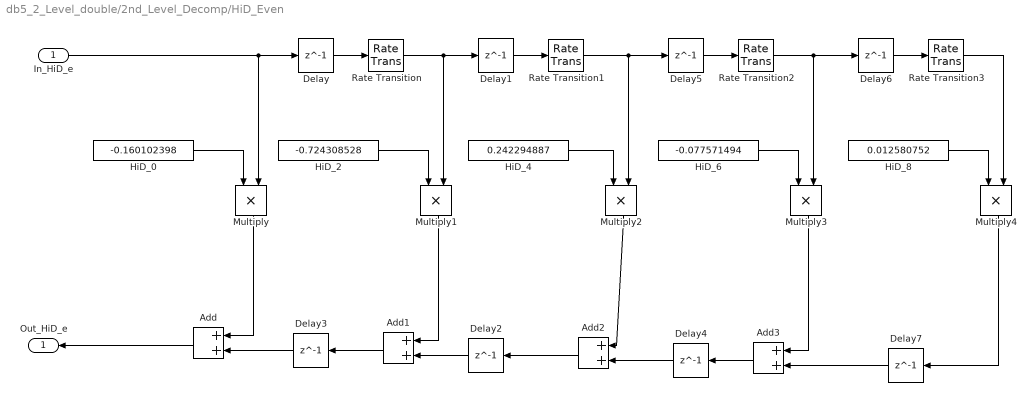
== system db5_2_Level_double/2nd_Level_Decomp/HiD_Even ==
  In_HiD_e : Inport  OutDataTypeStr=double  SampleTime=1/44100
  Add{,1..3} (4 alike) : Sum  AccumDataTypeStr=double  OutDataTypeStr=double
  Delay{,1..7} (8 alike) : Delay  DelayLength=1  SampleTime=1/44100
  HiD_0 : Constant  Value=-0.160102398  OutDataTypeStr=double  SampleTime=1/44100
  HiD_2 : Constant  Value=-0.724308528  OutDataTypeStr=double  SampleTime=1/44100
  HiD_4 : Constant  Value=0.242294887  OutDataTypeStr=double  SampleTime=1/44100
  HiD_6 : Constant  Value=-0.077571494  OutDataTypeStr=double  SampleTime=1/44100
  HiD_8 : Constant  Value=0.012580752  OutDataTypeStr=double  SampleTime=1/44100
  Multiply{,1..4} (5 alike) : Product  OutDataTypeStr=double
  Rate Transition{,1..3} (4 alike) : RateTransition  OutPortSampleTime=1/44100
  Out_HiD_e : Outport  OutDataTypeStr=double  SampleTime=1/44100  VectorParamsAs1DForOutWhenUnconnected=off
  wires:
  Delay1/1 -> Rate Transition1/1
  Delay3/1 -> Add/2
  HiD_2/1 -> Multiply1/1
  Rate Transition2/1 -> Delay6/1, Multiply3/2
  Add/1 -> Out_HiD_e/1
  Delay4/1 -> Add2/2
  Delay5/1 -> Rate Transition2/1
  Rate Transition1/1 -> Delay5/1, Multiply2/2
  HiD_0/1 -> Multiply/1
  Multiply2/1 -> Add2/1
  Add2/1 -> Delay2/1
  HiD_6/1 -> Multiply3/1
  Multiply/1 -> Add/1
  In_HiD_e/1 -> Delay/1, Multiply/2
  Multiply1/1 -> Add1/1
  Rate Transition/1 -> Delay1/1, Multiply1/2
  Add1/1 -> Delay3/1
  HiD_4/1 -> Multiply2/1
  Delay/1 -> Rate Transition/1
  Delay2/1 -> Add1/2
  HiD_8/1 -> Multiply4/1
  Delay6/1 -> Rate Transition3/1
  Rate Transition3/1 -> Multiply4/2
  Multiply4/1 -> Delay7/1
  Multiply3/1 -> Add3/1
  Add3/1 -> Delay4/1
  Delay7/1 -> Add3/2

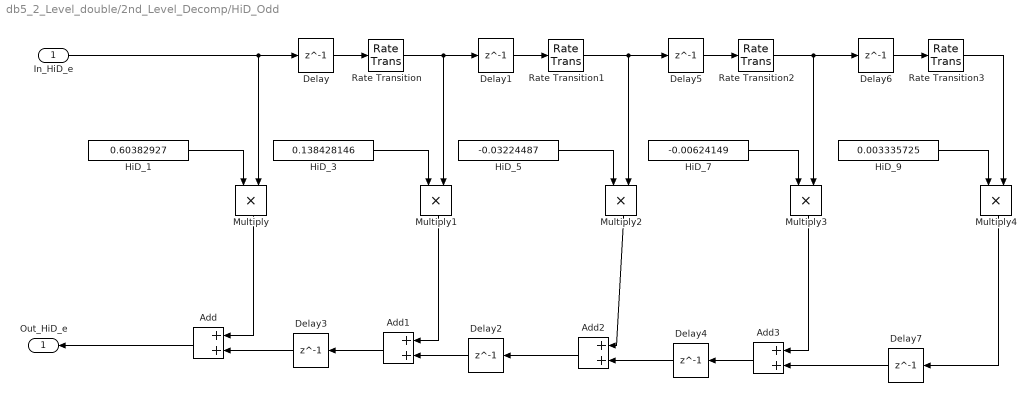
== system db5_2_Level_double/2nd_Level_Decomp/HiD_Odd ==
  In_HiD_e : Inport  OutDataTypeStr=double  SampleTime=1/44100
  Add{,1..3} (4 alike) : Sum  AccumDataTypeStr=double  OutDataTypeStr=double
  Delay{,1..7} (8 alike) : Delay  DelayLength=1  SampleTime=1/44100
  HiD_1 : Constant  Value=0.60382927  OutDataTypeStr=double  SampleTime=1/44100
  HiD_3 : Constant  Value=0.138428146  OutDataTypeStr=double  SampleTime=1/44100
  HiD_5 : Constant  Value=-0.03224487  OutDataTypeStr=double  SampleTime=1/44100
  HiD_7 : Constant  Value=-0.00624149  OutDataTypeStr=double  SampleTime=1/44100
  HiD_9 : Constant  Value=0.003335725  OutDataTypeStr=double  SampleTime=1/44100
  Multiply{,1..4} (5 alike) : Product  OutDataTypeStr=double
  Rate Transition{,1..3} (4 alike) : RateTransition  OutPortSampleTime=1/44100
  Out_HiD_e : Outport  OutDataTypeStr=double  SampleTime=1/44100  VectorParamsAs1DForOutWhenUnconnected=off
  wires:
  Multiply4/1 -> Delay7/1
  Delay6/1 -> Rate Transition3/1
  Rate Transition3/1 -> Multiply4/2
  Add3/1 -> Delay4/1
  Add/1 -> Out_HiD_e/1
  Delay1/1 -> Rate Transition1/1
  Delay7/1 -> Add3/2
  Rate Transition2/1 -> Delay6/1, Multiply3/2
  Delay3/1 -> Add/2
  Rate Transition/1 -> Delay1/1, Multiply1/2
  Rate Transition1/1 -> Delay5/1, Multiply2/2
  Delay4/1 -> Add2/2
  Multiply/1 -> Add/1
  Add2/1 -> Delay2/1
  Delay5/1 -> Rate Transition2/1
  Multiply1/1 -> Add1/1
  Delay2/1 -> Add1/2
  Delay/1 -> Rate Transition/1
  Add1/1 -> Delay3/1
  Multiply3/1 -> Add3/1
  HiD_3/1 -> Multiply1/1
  Multiply2/1 -> Add2/1
  HiD_7/1 -> Multiply3/1
  In_HiD_e/1 -> Delay/1, Multiply/2
  HiD_1/1 -> Multiply/1
  HiD_5/1 -> Multiply2/1
  HiD_9/1 -> Multiply4/1

== system db5_2_Level_double/2nd_Level_Decomp/LoD_Even ==
  In_HiD_e : Inport  OutDataTypeStr=double  SampleTime=1/44100
  Add{,1..3} (4 alike) : Sum  AccumDataTypeStr=double  OutDataTypeStr=double
  Delay{,1..7} (8 alike) : Delay  DelayLength=1  SampleTime=1/44100
  LoD_0 : Constant  Value=0.003335725  OutDataTypeStr=double  SampleTime=1/44100
  LoD_2 : Constant  Value=-0.00624149  OutDataTypeStr=double  SampleTime=1/44100
  LoD_4 : Constant  Value=-0.03224487  OutDataTypeStr=double  SampleTime=1/44100
  LoD_6 : Constant  Value=0.138428146  OutDataTypeStr=double  SampleTime=1/44100
  LoD_8 : Constant  Value=0.60382927  OutDataTypeStr=double  SampleTime=1/44100
  Multiply{,1..4} (5 alike) : Product  OutDataTypeStr=double
  Rate Transition{,1..3} (4 alike) : RateTransition  OutPortSampleTime=1/44100
  Out_HiD_e : Outport  OutDataTypeStr=double  SampleTime=1/44100  VectorParamsAs1DForOutWhenUnconnected=off
  wires:
  Multiply3/1 -> Add3/1
  LoD_4/1 -> Multiply2/1
  Multiply2/1 -> Add2/1
  Add1/1 -> Delay3/1
  Delay2/1 -> Add1/2
  Delay/1 -> Rate Transition/1
  Multiply1/1 -> Add1/1
  In_HiD_e/1 -> Delay/1, Multiply/2
  Add2/1 -> Delay2/1
  Delay5/1 -> Rate Transition2/1
  Multiply/1 -> Add/1
  LoD_8/1 -> Multiply4/1
  Delay4/1 -> Add2/2
  Rate Transition1/1 -> Delay5/1, Multiply2/2
  Rate Transition/1 -> Delay1/1, Multiply1/2
  Delay3/1 -> Add/2
  Rate Transition2/1 -> Delay6/1, Multiply3/2
  Add/1 -> Out_HiD_e/1
  Delay1/1 -> Rate Transition1/1
  Delay7/1 -> Add3/2
  LoD_6/1 -> Multiply3/1
  Add3/1 -> Delay4/1
  Rate Transition3/1 -> Multiply4/2
  Delay6/1 -> Rate Transition3/1
  Multiply4/1 -> Delay7/1
  LoD_2/1 -> Multiply1/1
  LoD_0/1 -> Multiply/1

== system db5_2_Level_double/2nd_Level_Decomp/LoD_Odd ==
  In_HiD_e : Inport  OutDataTypeStr=double  SampleTime=1/44100
  Add{,1..3} (4 alike) : Sum  AccumDataTypeStr=double  OutDataTypeStr=double
  Delay{,1..7} (8 alike) : Delay  DelayLength=1  SampleTime=1/44100
  LoD_1 : Constant  Value=-0.012580752  OutDataTypeStr=double  SampleTime=1/44100
  LoD_3 : Constant  Value=0.077571494  OutDataTypeStr=double  SampleTime=1/44100
  LoD_5 : Constant  Value=-0.242294887  OutDataTypeStr=double  SampleTime=1/44100
  LoD_7 : Constant  Value=0.724308528  OutDataTypeStr=double  SampleTime=1/44100
  LoD_9 : Constant  Value=0.160102398  OutDataTypeStr=double  SampleTime=1/44100
  Multiply{,1..4} (5 alike) : Product  OutDataTypeStr=double
  Rate Transition{,1..3} (4 alike) : RateTransition  OutPortSampleTime=1/44100
  Out_HiD_e : Outport  OutDataTypeStr=double  SampleTime=1/44100  VectorParamsAs1DForOutWhenUnconnected=off
  wires:
  LoD_9/1 -> Multiply4/1
  LoD_3/1 -> Multiply1/1
  LoD_5/1 -> Multiply2/1
  In_HiD_e/1 -> Delay/1, Multiply/2
  LoD_1/1 -> Multiply/1
  Multiply1/1 -> Add1/1
  Multiply3/1 -> Add3/1
  Multiply2/1 -> Add2/1
  Add1/1 -> Delay3/1
  Delay2/1 -> Add1/2
  Delay5/1 -> Rate Transition2/1
  Rate Transition/1 -> Delay1/1, Multiply1/2
  Multiply/1 -> Add/1
  Add2/1 -> Delay2/1
  Delay/1 -> Rate Transition/1
  Delay4/1 -> Add2/2
  Delay3/1 -> Add/2
  Delay7/1 -> Add3/2
  Add/1 -> Out_HiD_e/1
  Delay1/1 -> Rate Transition1/1
  Rate Transition2/1 -> Delay6/1, Multiply3/2
  Rate Transition1/1 -> Delay5/1, Multiply2/2
  LoD_7/1 -> Multiply3/1
  Multiply4/1 -> Delay7/1
  Delay6/1 -> Rate Transition3/1
  Add3/1 -> Delay4/1
  Rate Transition3/1 -> Multiply4/2

== system db5_2_Level_double/2nd_Level_Recon/HiR_Even ==
  In_HiR_e : Inport  OutDataTypeStr=double  SampleTime=1/44100
  Add{,1..3} (4 alike) : Sum  AccumDataTypeStr=double  OutDataTypeStr=double
  Delay{,1..7} (8 alike) : Delay  DelayLength=1  SampleTime=1/44100
  HiR_0 : Constant  Value=0.003335725  OutDataTypeStr=double  SampleTime=1/44100
  HiR_2 : Constant  Value=-0.00624149  OutDataTypeStr=double  SampleTime=1/44100
  HiR_4 : Constant  Value=-0.03224487  OutDataTypeStr=double  SampleTime=1/44100
  HiR_6 : Constant  Value=0.138428146  OutDataTypeStr=double  SampleTime=1/44100
  HiR_8 : Constant  Value=0.60382927  OutDataTypeStr=double  SampleTime=1/44100
  Multiply{,1..4} (5 alike) : Product  OutDataTypeStr=double
  Rate Transition{,1..3} (4 alike) : RateTransition  OutPortSampleTime=1/44100
  Out_HiR_e : Outport  OutDataTypeStr=double  SampleTime=1/44100  VectorParamsAs1DForOutWhenUnconnected=off
  wires:
  Delay3/1 -> Add/2
  In_HiR_e/1 -> Delay/1, Multiply/2
  HiR_4/1 -> Multiply2/1
  Multiply/1 -> Add/1
  Add1/1 -> Delay3/1
  Multiply1/1 -> Add1/1
  Delay2/1 -> Add1/2
  Add/1 -> Out_HiR_e/1
  HiR_0/1 -> Multiply/1
  HiR_2/1 -> Multiply1/1
  Delay1/1 -> Rate Transition1/1
  Rate Transition/1 -> Delay1/1, Multiply1/2
  Rate Transition1/1 -> Delay4/1, Multiply2/2
  Delay/1 -> Rate Transition/1
  Delay4/1 -> Rate Transition2/1
  HiR_6/1 -> Multiply3/1
  Multiply2/1 -> Add2/1
  Add2/1 -> Delay2/1
  Delay5/1 -> Add2/2
  Rate Transition3/1 -> Multiply4/2
  Multiply4/1 -> Delay7/1
  HiR_8/1 -> Multiply4/1
  Rate Transition2/1 -> Delay6/1, Multiply3/2
  Delay6/1 -> Rate Transition3/1
  Add3/1 -> Delay5/1
  Multiply3/1 -> Add3/1
  Delay7/1 -> Add3/2

== system db5_2_Level_double/2nd_Level_Recon/HiR_Odd ==
  In_HiR_o : Inport  OutDataTypeStr=double  SampleTime=1/44100
  Add{,1..3} (4 alike) : Sum  AccumDataTypeStr=double  OutDataTypeStr=double
  Delay{,1..7} (8 alike) : Delay  DelayLength=1  SampleTime=1/44100
  HiR_1 : Constant  Value=0.012580752  OutDataTypeStr=double  SampleTime=1/44100
  HiR_3 : Constant  Value=-0.077571494  OutDataTypeStr=double  SampleTime=1/44100
  HiR_5 : Constant  Value=0.242294887  OutDataTypeStr=double  SampleTime=1/44100
  HiR_7 : Constant  Value=-0.724308528  OutDataTypeStr=double  SampleTime=1/44100
  HiR_9 : Constant  Value=-0.160102398  OutDataTypeStr=double  SampleTime=1/44100
  Multiply{,1..4} (5 alike) : Product  OutDataTypeStr=double
  Rate Transition{,1..3} (4 alike) : RateTransition  OutPortSampleTime=1/44100
  Out_HiR_o : Outport  OutDataTypeStr=double  SampleTime=1/44100  VectorParamsAs1DForOutWhenUnconnected=off
  wires:
  Add/1 -> Out_HiR_o/1
  Add2/1 -> Delay2/1
  Delay5/1 -> Add2/2
  HiR_9/1 -> Multiply4/1
  HiR_5/1 -> Multiply2/1
  HiR_1/1 -> Multiply/1
  HiR_7/1 -> Multiply3/1
  Multiply1/1 -> Add1/1
  Multiply2/1 -> Add2/1
  Delay2/1 -> Add1/2
  Delay4/1 -> Rate Transition2/1
  Delay3/1 -> Add/2
  In_HiR_o/1 -> Delay/1, Multiply/2
  Rate Transition/1 -> Delay1/1, Multiply1/2
  Rate Transition2/1 -> Delay6/1, Multiply3/2
  Delay7/1 -> Add3/2
  Delay6/1 -> Rate Transition3/1
  Add3/1 -> Delay5/1
  Rate Transition3/1 -> Multiply4/2
  HiR_3/1 -> Multiply1/1
  Multiply3/1 -> Add3/1
  Add1/1 -> Delay3/1
  Multiply4/1 -> Delay7/1
  Multiply/1 -> Add/1
  Rate Transition1/1 -> Delay4/1, Multiply2/2
  Delay1/1 -> Rate Transition1/1
  Delay/1 -> Rate Transition/1

== system db5_2_Level_double/2nd_Level_Recon/LoR_Even ==
  In_LoR_e : Inport  OutDataTypeStr=double  SampleTime=1/44100
  Add{,1..3} (4 alike) : Sum  AccumDataTypeStr=double  OutDataTypeStr=double
  Delay{,1..7} (8 alike) : Delay  DelayLength=1  SampleTime=1/44100
  LoR_0 : Constant  Value=0.160102398  OutDataTypeStr=double  SampleTime=1/44100
  LoR_2 : Constant  Value=0.724308528  OutDataTypeStr=double  SampleTime=1/44100
  LoR_4 : Constant  Value=-0.242294887  OutDataTypeStr=double  SampleTime=1/44100
  LoR_6 : Constant  Value=0.077571494  OutDataTypeStr=double  SampleTime=1/44100
  LoR_8 : Constant  Value=-0.012580752  OutDataTypeStr=double  SampleTime=1/44100
  Multiply{,1..4} (5 alike) : Product  OutDataTypeStr=double
  Rate Transition{,1..3} (4 alike) : RateTransition  OutPortSampleTime=1/44100
  Out_LoR_e : Outport  OutDataTypeStr=double  SampleTime=1/44100  VectorParamsAs1DForOutWhenUnconnected=off
  wires:
  Add2/1 -> Delay2/1
  Delay5/1 -> Add2/2
  Add/1 -> Out_LoR_e/1
  Delay1/1 -> Rate Transition1/1
  Rate Transition1/1 -> Delay4/1, Multiply2/2
  Multiply/1 -> Add/1
  Add1/1 -> Delay3/1
  Delay/1 -> Rate Transition/1
  Multiply2/1 -> Add2/1
  Multiply1/1 -> Add1/1
  Delay3/1 -> Add/2
  Delay4/1 -> Rate Transition2/1
  Delay2/1 -> Add1/2
  Rate Transition/1 -> Delay1/1, Multiply1/2
  In_LoR_e/1 -> Delay/1, Multiply/2
  LoR_4/1 -> Multiply2/1
  Delay6/1 -> Rate Transition3/1
  LoR_0/1 -> Multiply/1
  Delay7/1 -> Add3/2
  Rate Transition2/1 -> Delay6/1, Multiply3/2
  LoR_8/1 -> Multiply4/1
  LoR_2/1 -> Multiply1/1
  Rate Transition3/1 -> Multiply4/2
  LoR_6/1 -> Multiply3/1
  Multiply4/1 -> Delay7/1
  Multiply3/1 -> Add3/1
  Add3/1 -> Delay5/1

== system db5_2_Level_double/2nd_Level_Recon/LoR_Odd ==
  In_LoR_o : Inport  OutDataTypeStr=double  SampleTime=1/44100
  Add{,1..3} (4 alike) : Sum  AccumDataTypeStr=double  OutDataTypeStr=double
  Delay{,1..7} (8 alike) : Delay  DelayLength=1  SampleTime=1/44100
  LoR_1 : Constant  Value=0.60382927  OutDataTypeStr=double  SampleTime=1/44100
  LoR_3 : Constant  Value=0.138428146  OutDataTypeStr=double  SampleTime=1/44100
  LoR_5 : Constant  Value=-0.03224487  OutDataTypeStr=double  SampleTime=1/44100
  LoR_7 : Constant  Value=-0.00624149  OutDataTypeStr=double  SampleTime=1/44100
  LoR_9 : Constant  Value=0.003335725  OutDataTypeStr=double  SampleTime=1/44100
  Multiply{,1..4} (5 alike) : Product  OutDataTypeStr=double
  Rate Transition{,1..3} (4 alike) : RateTransition  OutPortSampleTime=1/44100
  Out_LoR_o : Outport  OutDataTypeStr=double  SampleTime=1/44100  VectorParamsAs1DForOutWhenUnconnected=off
  wires:
  LoR_9/1 -> Multiply4/1
  Rate Transition2/1 -> Delay6/1, Multiply3/2
  Rate Transition/1 -> Delay1/1, Multiply1/2
  Rate Transition3/1 -> Multiply4/2
  Add3/1 -> Delay5/1
  Delay6/1 -> Rate Transition3/1
  Delay7/1 -> Add3/2
  LoR_1/1 -> Multiply/1
  LoR_3/1 -> Multiply1/1
  Delay3/1 -> Add/2
  Delay4/1 -> Rate Transition2/1
  LoR_5/1 -> Multiply2/1
  Delay2/1 -> Add1/2
  Multiply2/1 -> Add2/1
  Add2/1 -> Delay2/1
  LoR_7/1 -> Multiply3/1
  Delay5/1 -> Add2/2
  Multiply3/1 -> Add3/1
  Multiply/1 -> Add/1
  Delay1/1 -> Rate Transition1/1
  Multiply4/1 -> Delay7/1
  In_LoR_o/1 -> Delay/1, Multiply/2
  Add1/1 -> Delay3/1
  Add/1 -> Out_LoR_o/1
  Rate Transition1/1 -> Delay4/1, Multiply2/2
  Delay/1 -> Rate Transition/1
  Multiply1/1 -> Add1/1

== system db5_2_Level_double/Threshold_Estimator/Absolute_Value1 ==
  Signal_w4 : Inport  OutDataTypeStr=double  SampleTime=1/44100
  Absolute_Switch : Switch  Threshold=1  OutDataTypeStr=double
  Constant295 : Constant  Value=0  OutDataTypeStr=double  SampleTime=1/44100
  Gain2 : Gain  Gain=-1  ParamDataTypeStr=double  OutDataTypeStr=double
  Relational Operator2 : RelationalOperator  Operator=<  OutDataTypeStr=boolean  RndMeth=Simplest
  Out_Abs : Outport  OutDataTypeStr=double  SampleTime=1/44100  VectorParamsAs1DForOutWhenUnconnected=off
  wires:
  Absolute_Switch/1 -> Out_Abs/1
  Relational Operator2/1 -> Absolute_Switch/2
  Gain2/1 -> Absolute_Switch/1
  Signal_w4/1 -> Absolute_Switch/3, Relational Operator2/1, Gain2/1
  Constant295/1 -> Relational Operator2/2

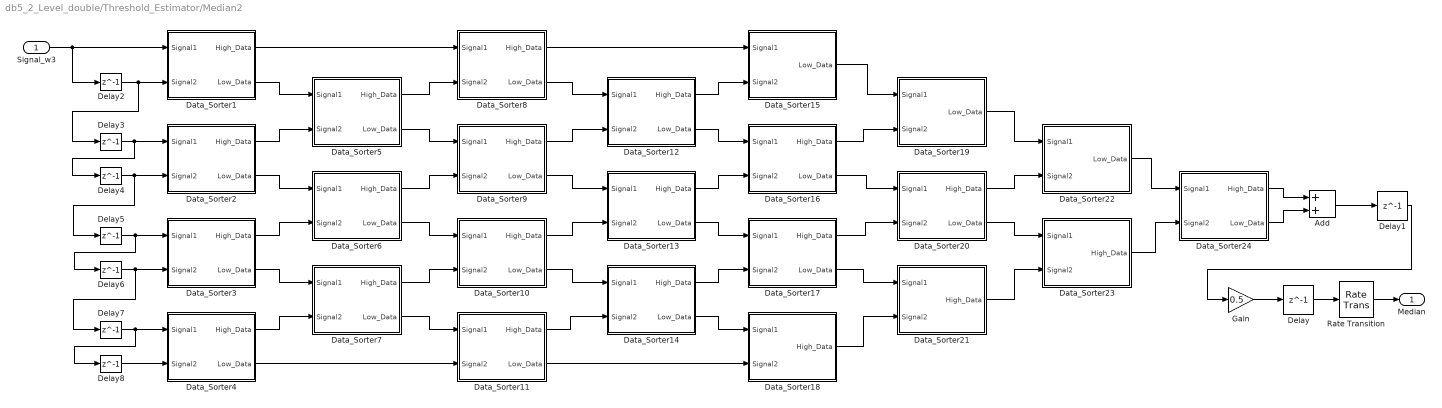
== system db5_2_Level_double/Threshold_Estimator/Median2 ==
  Signal_w3 : Inport  OutDataTypeStr=double  SampleTime=1/44100
  Add : Sum  AccumDataTypeStr=double  OutDataTypeStr=double  LockScale=on
  Data_Sorter1 : Subsystem
  Data_Sorter10 : Subsystem
  Data_Sorter11 : Subsystem
  Data_Sorter12 : Subsystem
  Data_Sorter13 : Subsystem
  Data_Sorter14 : Subsystem
  Data_Sorter15 : Subsystem
  Data_Sorter16 : Subsystem
  Data_Sorter17 : Subsystem
  Data_Sorter18 : Subsystem
  Data_Sorter19 : Subsystem
  Data_Sorter2 : Subsystem
  Data_Sorter20 : Subsystem
  Data_Sorter21 : Subsystem
  Data_Sorter22 : Subsystem
  Data_Sorter23 : Subsystem
  Data_Sorter24 : Subsystem
  Data_Sorter3 : Subsystem
  Data_Sorter4 : Subsystem
  Data_Sorter5 : Subsystem
  Data_Sorter6 : Subsystem
  Data_Sorter7 : Subsystem
  Data_Sorter8 : Subsystem
  Data_Sorter9 : Subsystem
  Delay{,1..8} (9 alike) : Delay  DelayLength=1  SampleTime=1/44100
  Gain : Gain  Gain=0.5  ParamDataTypeStr=double  OutDataTypeStr=double
  Rate Transition : RateTransition  OutPortSampleTime=1/44100
  Median : Outport  OutDataTypeStr=double  SampleTime=1/44100  VectorParamsAs1DForOutWhenUnconnected=off
  wires:
  Data_Sorter4/1(High_Data) -> Data_Sorter7/2(Signal2)
  Delay3/1 -> Data_Sorter2/1(Signal1), Delay4/1
  Signal_w3/1 -> Data_Sorter1/1(Signal1), Delay2/1
  Data_Sorter10/1(High_Data) -> Data_Sorter13/2(Signal2)
  Data_Sorter23/1(High_Data) -> Data_Sorter24/2(Signal2)
  Data_Sorter12/2(Low_Data) -> Data_Sorter16/1(Signal1)
  Delay2/1 -> Delay3/1, Data_Sorter1/2(Signal2)
  Data_Sorter5/1(High_Data) -> Data_Sorter8/2(Signal2)
  Delay/1 -> Rate Transition/1
  Data_Sorter15/1(Low_Data) -> Data_Sorter19/1(Signal1)
  Add/1 -> Delay1/1
  Data_Sorter7/2(Low_Data) -> Data_Sorter11/1(Signal1)
  Data_Sorter24/1(High_Data) -> Add/1
  Data_Sorter1/2(Low_Data) -> Data_Sorter5/1(Signal1)
  Data_Sorter3/1(High_Data) -> Data_Sorter6/2(Signal2)
  Data_Sorter22/1(Low_Data) -> Data_Sorter24/1(Signal1)
  Data_Sorter2/1(High_Data) -> Data_Sorter5/2(Signal2)
  Data_Sorter10/2(Low_Data) -> Data_Sorter14/1(Signal1)
  Delay1/1 -> Gain/1
  Data_Sorter17/2(Low_Data) -> Data_Sorter21/1(Signal1)
  Data_Sorter21/1(High_Data) -> Data_Sorter23/2(Signal2)
  Data_Sorter7/1(High_Data) -> Data_Sorter10/2(Signal2)
  Delay4/1 -> Data_Sorter2/2(Signal2), Delay5/1
  Data_Sorter16/1(High_Data) -> Data_Sorter19/2(Signal2)
  Data_Sorter20/1(High_Data) -> Data_Sorter22/2(Signal2)
  Data_Sorter16/2(Low_Data) -> Data_Sorter20/1(Signal1)
  Data_Sorter3/2(Low_Data) -> Data_Sorter7/1(Signal1)
  Data_Sorter2/2(Low_Data) -> Data_Sorter6/1(Signal1)
  Data_Sorter6/2(Low_Data) -> Data_Sorter10/1(Signal1)
  Data_Sorter19/1(Low_Data) -> Data_Sorter22/1(Signal1)
  Data_Sorter12/1(High_Data) -> Data_Sorter15/2(Signal2)
  Data_Sorter5/2(Low_Data) -> Data_Sorter9/1(Signal1)
  Data_Sorter24/2(Low_Data) -> Add/2
  Data_Sorter17/1(High_Data) -> Data_Sorter20/2(Signal2)
  Data_Sorter13/1(High_Data) -> Data_Sorter16/2(Signal2)
  Data_Sorter11/1(High_Data) -> Data_Sorter14/2(Signal2)
  Delay8/1 -> Data_Sorter4/2(Signal2)
  Data_Sorter8/2(Low_Data) -> Data_Sorter12/1(Signal1)
  Delay6/1 -> Data_Sorter3/2(Signal2), Delay7/1
  Data_Sorter9/2(Low_Data) -> Data_Sorter13/1(Signal1)
  Data_Sorter4/2(Low_Data) -> Data_Sorter11/2(Signal2)
  Data_Sorter9/1(High_Data) -> Data_Sorter12/2(Signal2)
  Data_Sorter14/2(Low_Data) -> Data_Sorter18/1(Signal1)
  Delay5/1 -> Data_Sorter3/1(Signal1), Delay6/1
  Delay7/1 -> Data_Sorter4/1(Signal1), Delay8/1
  Data_Sorter1/1(High_Data) -> Data_Sorter8/1(Signal1)
  Data_Sorter8/1(High_Data) -> Data_Sorter15/1(Signal1)
  Data_Sorter14/1(High_Data) -> Data_Sorter17/2(Signal2)
  Data_Sorter6/1(High_Data) -> Data_Sorter9/2(Signal2)
  Data_Sorter20/2(Low_Data) -> Data_Sorter23/1(Signal1)
  Data_Sorter11/2(Low_Data) -> Data_Sorter18/2(Signal2)
  Data_Sorter13/2(Low_Data) -> Data_Sorter17/1(Signal1)
  Gain/1 -> Delay/1
  Data_Sorter18/1(High_Data) -> Data_Sorter21/2(Signal2)
  Rate Transition/1 -> Median/1

== system db5_2_Level_double/Threshold_Estimator/Median2/Data_Sorter1 ==
  Signal1 : Inport  OutDataTypeStr=double  SampleTime=1/44100
  Signal2 : Inport  Port=2  OutDataTypeStr=double  SampleTime=1/44100
  Data_Sorter_Switch : Switch  OutDataTypeStr=double
  Data_Sorter_Switch1 : Switch  Threshold=1  OutDataTypeStr=double
  Delay1 : Delay  DelayLength=1  SampleTime=1/44100
  Delay2 : Delay  DelayLength=1  SampleTime=1/44100
  Relational Operator2 : RelationalOperator  Operator=<  OutDataTypeStr=boolean  RndMeth=Simplest
  High_Data : Outport  OutDataTypeStr=double  SampleTime=1/44100  VectorParamsAs1DForOutWhenUnconnected=off
  Low_Data : Outport  Port=2  OutDataTypeStr=double  SampleTime=1/44100  VectorParamsAs1DForOutWhenUnconnected=off
  wires:
  Signal1/1 -> Data_Sorter_Switch/3, Data_Sorter_Switch/1, Relational Operator2/1
  Relational Operator2/1 -> Data_Sorter_Switch1/2, Data_Sorter_Switch/2
  Signal2/1 -> Data_Sorter_Switch1/1, Data_Sorter_Switch1/3, Relational Operator2/2
  Data_Sorter_Switch1/1 -> Delay2/1
  Delay2/1 -> Low_Data/1
  Data_Sorter_Switch/1 -> Delay1/1
  Delay1/1 -> High_Data/1
